simulink model "linetrack"  (Simulink 7.3)
settings: Solver=ode45  StartTime=0.0  StopTime=6  RelTol=1e-3
libraries: simulink x1
settings Model: Creator=Sainquake  LastModifiedBy=Sainquake

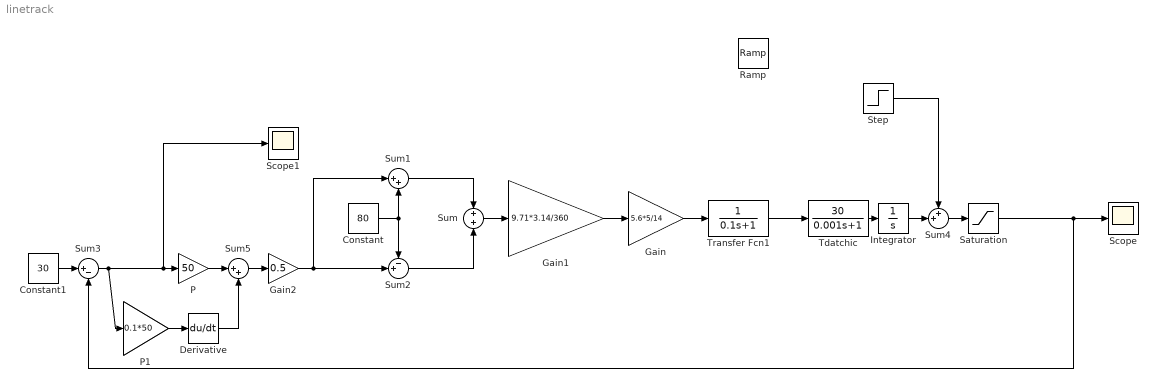
== system linetrack ==
  Constant : Constant  Value=80  OutDataType=fixdt(1, 16)  OutScaling=2^0
  Constant1 : Constant  Value=30  OutDataType=fixdt(1, 16)  OutScaling=2^0
  Derivative : Derivative
  Gain : Gain  Gain=5.6*5/14  ParameterDataType=fixdt(1, 16)  ParameterScaling=2^0  OutDataType=fixdt(1, 16)  OutScaling=2^0
  Gain1 : Gain  Gain=9.71*3.14/360  ParameterDataType=fixdt(1, 16)  ParameterScaling=2^0  OutDataType=fixdt(1, 16)  OutScaling=2^0
  Gain2 : Gain  Gain=0.5  ParameterDataType=fixdt(1, 16)  ParameterScaling=2^0  OutDataType=fixdt(1, 16)  OutScaling=2^0
  Integrator : Integrator
  P : Gain  Gain=50  ParameterDataType=fixdt(1, 16)  ParameterScaling=2^0  OutDataType=fixdt(1, 16)  OutScaling=2^0
  P1 : Gain  Gain=0.1*50  ParameterDataType=fixdt(1, 16)  ParameterScaling=2^0  OutDataType=fixdt(1, 16)  OutScaling=2^0
  Ramp : simulink/Sources/Ramp  SystemSampleTime=-1  slope=10  start=0  X0=0
  Saturation : Saturate  UpperLimit=40  LowerLimit=20  OutDataType=fixdt(1, 16)  OutScaling=2^0
  Scope : Scope
  Scope1 : Scope
  Step : Step  Time=3  After=20  SampleTime=0
  Sum : Sum  Inputs=+|+  OutDataType=fixdt(1, 16)  OutScaling=2^0
  Sum1 : Sum  Inputs=|++  OutDataType=fixdt(1, 16)  OutScaling=2^0
  Sum2 : Sum  Inputs=-+|  OutDataType=fixdt(1, 16)  OutScaling=2^0
  Sum3 : Sum  Inputs=|+-  OutDataType=fixdt(1, 16)  OutScaling=2^0
  Sum4 : Sum  Inputs=++|  OutDataType=fixdt(1, 16)  OutScaling=2^0
  Sum5 : Sum  Inputs=|++  OutDataType=fixdt(1, 16)  OutScaling=2^0
  Tdatchic : TransferFcn  Numerator=[30]  Denominator=[0.001 1]
  Transfer Fcn1 : TransferFcn  Denominator=[0.1 1]
  wires:
  Transfer Fcn1/1 -> Tdatchic/1
  Tdatchic/1 -> Integrator/1
  Sum/1 -> Gain1/1
  Gain1/1 -> Gain/1
  Constant/1 -> Sum2/1, Sum1/2
  Sum1/1 -> Sum/1
  Sum2/1 -> Sum/2
  Gain2/1 -> Sum2/2, Sum1/1
  Constant1/1 -> Sum3/1
  Sum3/1 -> Scope1/1, P/1, P1/1
  Gain/1 -> Transfer Fcn1/1
  P/1 -> Sum5/1
  Step/1 -> Sum4/1
  Saturation/1 -> Scope/1, Sum3/2
  Sum4/1 -> Saturation/1
  Integrator/1 -> Sum4/2
  Sum5/1 -> Gain2/1
  Derivative/1 -> Sum5/2
  P1/1 -> Derivative/1
